simulink model "ex2p1"  (R2016b)
settings: Solver=VariableStepAuto  StartTime=0.0  StopTime=0.1  RelTol=1e-3
InitFcn:
  | alpha = 60;
libraries: powerlib x7, simulink x2
settings Model: Creator=user  LastModifiedBy=user

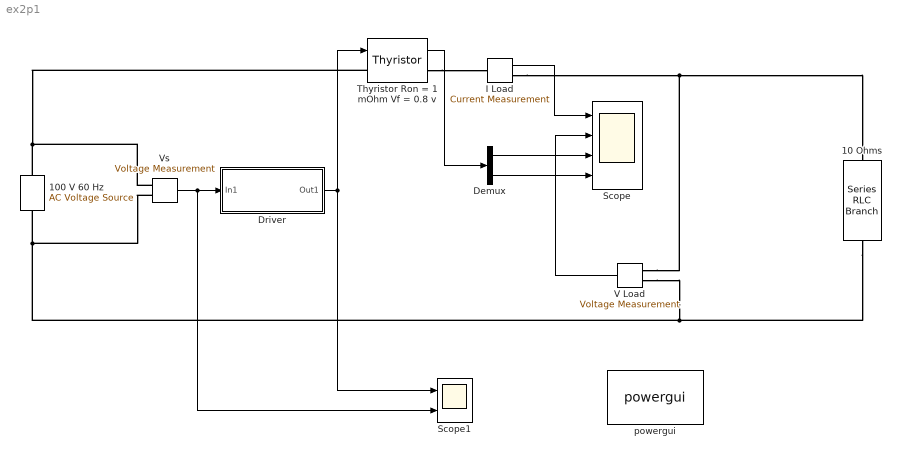
== system ex2p1 ==
  "10 Ohms " : powerlib/Elements/Series RLC Branch  LConnTagsString=__new0  RConnTagsString=__new0  BranchType=R  Resistance=10  Inductance=10e-3  SetiL0=off  InitialCurrent=0  Capacitance=1e-6  Setx0=off  InitialVoltage=0  Measurements=None
  100 V 60 Hz : powerlib/Electrical Sources/AC Voltage Source  Amplitude=100  Phase=0  Frequency=60  SampleTime=0  Measurements=None  BusType=swing  Pref=10e3  Qref=0  Qmin=-inf  Qmax=+inf
  Demux : Demux  Outputs=2
  Driver : Subsystem
  I Load : powerlib/Measurements/Current Measurement  PhasorSimulation=off  OutputType=Complex  PSBequivalent=0
  Scope : Scope  NumInputPorts=4
  Scope1 : Scope  NumInputPorts=2
  Thyristor Ron = 1 mOhm Vf = 0.8 v : powerlib/Power Electronics/Thyristor  Ron=0.001  Lon=0  Vf=0.8  IC=0  Rs=500  Cs=250e-9  Measurements=on
  V Load : powerlib/Measurements/Voltage Measurement  PhasorSimulation=off  OutputType=Complex  PSBequivalent=0
  Vs : powerlib/Measurements/Voltage Measurement  PhasorSimulation=off  OutputType=Complex  PSBequivalent=0
  powergui : powerlib/powergui  Priority=1  SimulationMode=Continuous  SolverType=Tustin/Backward Euler (TBE)  SampleTime=50e-6  frequency=60  SPID=off  DisableSnubberDevices=off  DisableRonSwitches=off  DisableVfSwitches=off  SwTol=0  DisplayEquations=off  Interpol=off  ExternalGateDelay=off  methode=off  Ts=10  FunctionMessages=off  echomessages=off  HookPort=off  EnableUseOfTLC=off  x0status=blocks  frequencyindice=60  Pbase=100e6  ErrMax=1e-4  Iterations=50  UnitsV=kV  UnitsW=MW  buscounter=0  RestoreLinks=warning  ResistiveCurrentMeasurement=off  Frange=[0:2:500]  Ylog=off  Xlog=on  ShowGrid=off  save=off  variable=ZData  structure=0  ZoomFFT=off  StartTime=0.0  cycles=1  DisplayStyle=1  fundamental=60  FreqAxis=off  MaxFrequency=1000  frequencyindicesteady=1  RmsSteady=1  display=off
  wires:
  Vs/1 -> Scope1/2, Driver/1(In1)
  Driver/1(Out1) -> Thyristor Ron = 1 mOhm Vf = 0.8 v/1, Scope1/1
  I Load/1 -> Scope/1
  Thyristor Ron = 1 mOhm Vf = 0.8 v/1 -> Demux/1
  Demux/1 -> Scope/3
  Demux/2 -> Scope/4
  V Load/1 -> Scope/2
  connections:
  100 V 60 Hz/RConn1 -- Thyristor Ron = 1 mOhm Vf = 0.8 v/LConn1 -- Vs/LConn1
  "10 Ohms "/RConn1 -- V Load/LConn2 -- Vs/LConn2 -- 100 V 60 Hz/LConn1
  Thyristor Ron = 1 mOhm Vf = 0.8 v/RConn1 -- I Load/LConn1
  I Load/RConn1 -- V Load/LConn1 -- "10 Ohms "/LConn1

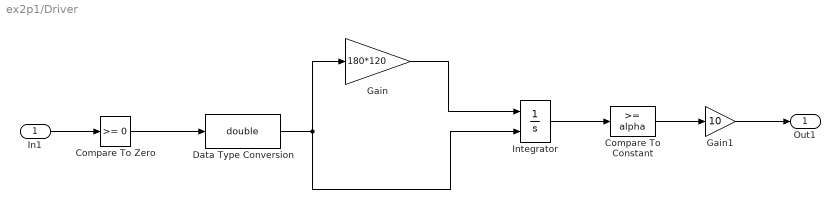
== system ex2p1/Driver ==
  In1 : Inport
  Compare To Constant : simulink/Logic and Bit Operations/Compare To Constant  relop=>=  const=alpha  OutDataTypeStr=boolean
  Compare To Zero : simulink/Logic and Bit Operations/Compare To Zero  relop=>=  OutDataTypeStr=boolean
  Data Type Conversion : DataTypeConversion  OutDataTypeStr=double
  Gain : Gain  Gain=180*120
  Gain1 : Gain  Gain=10
  Integrator : Integrator  ExternalReset=falling
  Out1 : Outport
  wires:
  In1/1 -> Compare To Zero/1
  Compare To Zero/1 -> Data Type Conversion/1
  Gain/1 -> Integrator/1
  Data Type Conversion/1 -> Gain/1, Integrator/2
  Integrator/1 -> Compare To Constant/1
  Compare To Constant/1 -> Gain1/1
  Gain1/1 -> Out1/1
